simulink library "BLDC"  (Simulink 8.0)
settings: Solver=ode45  StartTime=0.0  StopTime=10.0  RelTol=1e-3
libraries: simulink x18, BLDC x1
settings Model: Creator=Juliano  LastModifiedBy=h3now

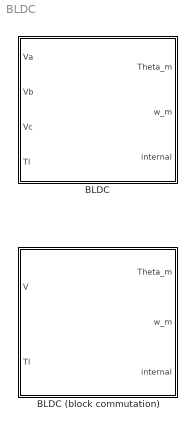
== system BLDC ==
  BLDC : Subsystem  mask(Simulador de um motor BLDC){J=1.39e-6, R=10.1/2, L=2.04/2000, P=8, Kt=15.7e-3/1.19, Ke=15.7e-3/1.19, Kd=0}
      mask prompts: J "Inércia do sistema motor+carga [Kg.m^2]"; R "Resistência por fase [Ohm]"; L "Indutância por fase [Henry]"; P "Número de pólos"; Kt "Constante de torque [Nm/A]"; Ke "Constante de força eletromotriz [V.s] (numericamente igual à constante de torque se utilizar SI)"; Kd "Constante de atrito viscoso"
      mask help:
      | Entradas
      | - Vx: tensões na fase 'x' [V]
      | - Tl: torque da carga [N.m]
      |
      | Saídas
      | - Theta_m: ângulo do rotor [rad]
      | - w_m: velocidade ângular do rotor [rad/s]
      | - internal: vetor de variáveis internas do simulador:
      |     - FCEM em cada fase [V] (3x1)
      |     - Corrente em cada fase [A] (3x1)
      |     - Torque produzido por cada fase [N.m] (3x1)
      |     - Torque total [N.m] (1x1)
  BLDC (block commutation) : Subsystem  mask(Simulador BLDC (block commutation)){J=1.39e-6, R=10.1/2, L=2.04/2000, P=8, Kt=15.7e-3/1.19, Ke=15.7e-3/1.19, Kd=0}
      mask prompts: J "Inércia do motor [Kg.m^2]"; R "Resistência por fase [Ohm]"; L "Indutância por fase [Henry]"; P "Número de pólos"; Kt "Constante de torque [Nm/A]"; Ke "Constante de força eletromotriz [V.s] (numericamente igual à constante de torque se SI)"; Kd "Constante de atrito viscoso"
      mask help:
      | Entradas
      | - Vx: tensões na fase 'x' [V]
      | - Tl: torque da carga [N.m]
      |
      | Saídas
      | - Theta_m: ângulo do rotor [rad]
      | - w_m: velocidade ângular do rotor [rad/s]
      | - internal: vetor de variáveis internas do simulador:
      |     - FCEM em cada fase [V] (3x1)
      |     - Corrente em cada fase [A] (3x1)
      |     - Torque produzido por cada fase [N.m] (3x1)
      |     - Torque total [N.m] (1x1)
      mask TypeOptions J: BLDC/J
      mask TypeOptions R: BLDC/R
      mask TypeOptions L: BLDC/L
      mask TypeOptions P: BLDC/P
      mask TypeOptions Kt: BLDC/Kt
      mask TypeOptions Ke: BLDC/Ke
      mask TypeOptions Kd: BLDC/Kd

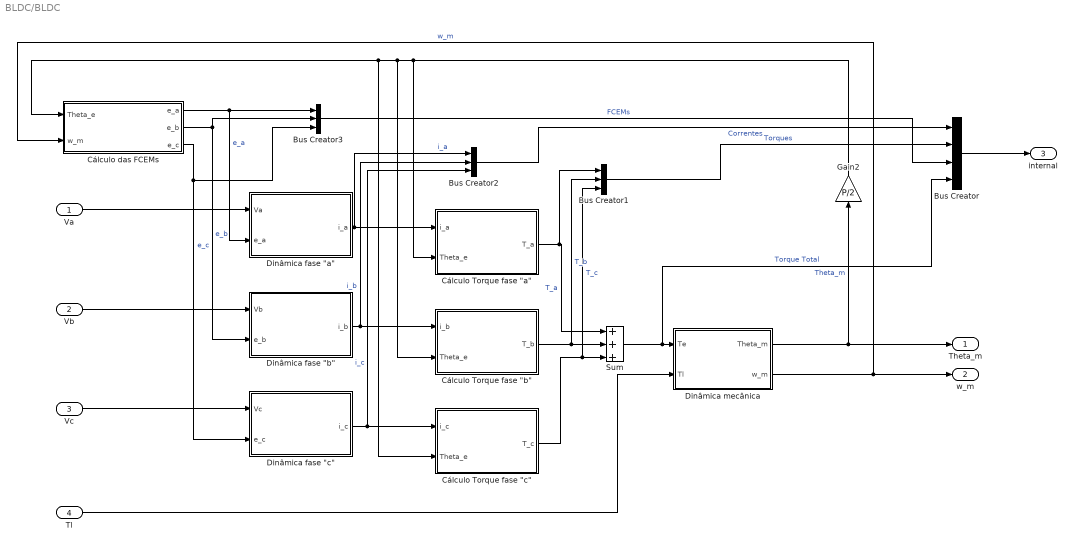
== system BLDC/BLDC ==
  Va : Inport
  Vb : Inport  Port=2
  Vc : Inport  Port=3
  Tl : Inport  Port=4
  Bus Creator : BusCreator
  Bus Creator1 : BusCreator  Inputs=3
  Bus Creator2 : BusCreator  Inputs=3
  Bus Creator3 : BusCreator  Inputs=3
  "Cálculo Torque fase \"a\"" : Subsystem
  "Cálculo Torque fase \"b\"" : Subsystem
  "Cálculo Torque fase \"c\"" : Subsystem
  Cálculo das FCEMs : Subsystem
  "Dinâmica fase \"a\"" : Subsystem
  "Dinâmica fase \"b\"" : Subsystem
  "Dinâmica fase \"c\"" : Subsystem
  "Dinâmica mecânica " : Subsystem
  Gain2 : Gain  Gain=P/2
  Sum : Sum  Inputs=+++
  Theta_m : Outport
  w_m : Outport  Port=2
  internal : Outport  Port=3
  wires:
  Gain2/1 -> "Cálculo Torque fase \"b\""/2(Theta_e), Cálculo das FCEMs/1(Theta_e), "Cálculo Torque fase \"c\""/2(Theta_e), "Cálculo Torque fase \"a\""/2(Theta_e)
  Tl/1 -> "Dinâmica mecânica "/2(Tl)
  "Dinâmica mecânica "/2(w_m) -> w_m/1, Cálculo das FCEMs/2(w_m)  "w_m"
  "Dinâmica mecânica "/1(Theta_m) -> Gain2/1, Theta_m/1  "Theta_m"
  Sum/1 -> Bus Creator/4, "Dinâmica mecânica "/1(Te)  "Torque Total"
  "Cálculo Torque fase \"c\""/1(T_c) -> Bus Creator1/3, Sum/3  "T_c"
  "Cálculo Torque fase \"b\""/1(T_b) -> Bus Creator1/2, Sum/2  "T_b"
  "Cálculo Torque fase \"a\""/1(T_a) -> Bus Creator1/1, Sum/1  "T_a"
  "Dinâmica fase \"c\""/1(i_c) -> Bus Creator2/3, "Cálculo Torque fase \"c\""/1(i_c)  "i_c"
  "Dinâmica fase \"b\""/1(i_b) -> Bus Creator2/2, "Cálculo Torque fase \"b\""/1(i_b)  "i_b"
  "Dinâmica fase \"a\""/1(i_a) -> Bus Creator2/1, "Cálculo Torque fase \"a\""/1(i_a)  "i_a"
  Vc/1 -> "Dinâmica fase \"c\""/1(Vc)
  Vb/1 -> "Dinâmica fase \"b\""/1(Vb)
  Va/1 -> "Dinâmica fase \"a\""/1(Va)
  Cálculo das FCEMs/3(e_c) -> Bus Creator3/3, "Dinâmica fase \"c\""/2(e_c)  "e_c"
  Cálculo das FCEMs/2(e_b) -> Bus Creator3/2, "Dinâmica fase \"b\""/2(e_b)  "e_b"
  Cálculo das FCEMs/1(e_a) -> Bus Creator3/1, "Dinâmica fase \"a\""/2(e_a)  "e_a"
  Bus Creator/1 -> internal/1
  Bus Creator3/1 -> Bus Creator/3  "FCEMs"
  Bus Creator2/1 -> Bus Creator/1  "Correntes"
  Bus Creator1/1 -> Bus Creator/2  "Torques"

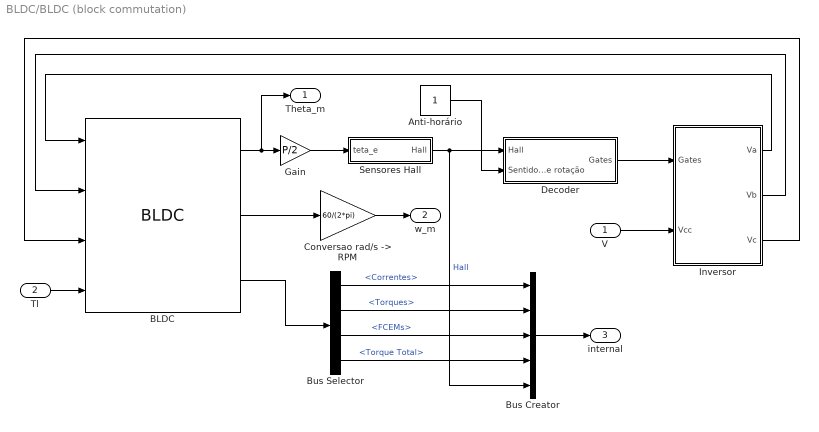
== system BLDC/BLDC (block commutation) ==
  V : Inport
  Tl : Inport  Port=2
  Anti-horário : Constant
  BLDC : BLDC/BLDC  J=J  R=R  L=L  P=P  Kt=Kt  Ke=Ke  Kd=Kd
  Bus Creator : BusCreator  Inputs=5
  Bus Selector : BusSelector  OutputSignals=Correntes,Torques,FCEMs,Torque Total
  "Conversao rad/s -> RPM" : Gain  Gain=60/(2*pi)
  Decoder : Subsystem
  Gain : Gain  Gain=P/2
  Inversor : Subsystem
  Sensores Hall : Subsystem  AncestorBlock=spsPMSynchronousMachineModel/Discrete Trapezoidal/Hall effect sensor
  Theta_m : Outport
  w_m : Outport  Port=2
  internal : Outport  Port=3
  wires:
  BLDC/1 -> Theta_m/1, Gain/1
  Gain/1 -> Sensores Hall/1(teta_e)
  Decoder/1(Gates) -> Inversor/1(Gates)
  Anti-horário/1 -> Decoder/2(Sentido de rotação)
  Tl/1 -> BLDC/4
  Inversor/1(Va) -> BLDC/1
  Inversor/2(Vb) -> BLDC/2
  Inversor/3(Vc) -> BLDC/3
  BLDC/2 -> "Conversao rad/s -> RPM"/1
  "Conversao rad/s -> RPM"/1 -> w_m/1
  V/1 -> Inversor/2(Vcc)
  Sensores Hall/1(Hall) -> Bus Creator/5, Decoder/1("Hall ")  "Hall"
  BLDC/3 -> Bus Selector/1
  Bus Selector/1 -> Bus Creator/1  "<Correntes>"
  Bus Selector/2 -> Bus Creator/2  "<Torques>"
  Bus Selector/3 -> Bus Creator/3  "<FCEMs>"
  Bus Selector/4 -> Bus Creator/4  "<Torque Total>"
  Bus Creator/1 -> internal/1

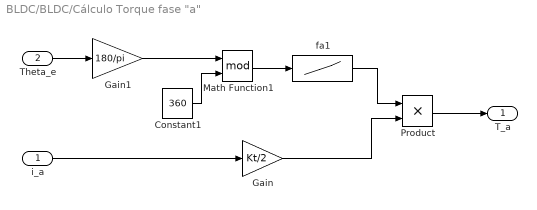
== system BLDC/BLDC/Cálculo Torque fase "a" ==
  i_a : Inport
  Theta_e : Inport  Port=2
  Constant1 : Constant  Value=360
  Gain : Gain  Gain=Kt/2
  Gain1 : Gain  Gain=180/pi
  Math Function1 : Math  Operator=mod  SaturateOnIntegerOverflow=on
  Product : Product  RndMeth=Zero
  fa1 : Lookup  InputValues=[0 30 60 90 120 150 180 210 240 270 300 330 360]  Table=[ 1 1 1 0 -1 -1 -1 -1 -1 0 1 1 1]
  T_a : Outport
  wires:
  Constant1/1 -> Math Function1/2
  Gain1/1 -> Math Function1/1
  Product/1 -> T_a/1
  fa1/1 -> Product/1
  Theta_e/1 -> Gain1/1
  Math Function1/1 -> fa1/1
  Gain/1 -> Product/2
  i_a/1 -> Gain/1

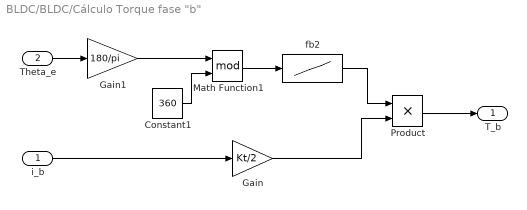
== system BLDC/BLDC/Cálculo Torque fase "b" ==
  i_b : Inport
  Theta_e : Inport  Port=2
  Constant1 : Constant  Value=360
  Gain : Gain  Gain=Kt/2
  Gain1 : Gain  Gain=180/pi
  Math Function1 : Math  Operator=mod  SaturateOnIntegerOverflow=on
  Product : Product  RndMeth=Zero
  fb2 : Lookup  InputValues=[0 30 60 90 120 150 180 210 240 270 300 330 360]  Table=[-1 0 1 1 1 1 1 0 -1 -1 -1 -1 -1]
  T_b : Outport
  wires:
  Constant1/1 -> Math Function1/2
  Gain1/1 -> Math Function1/1
  i_b/1 -> Gain/1
  Gain/1 -> Product/2
  Math Function1/1 -> fb2/1
  Theta_e/1 -> Gain1/1
  fb2/1 -> Product/1
  Product/1 -> T_b/1

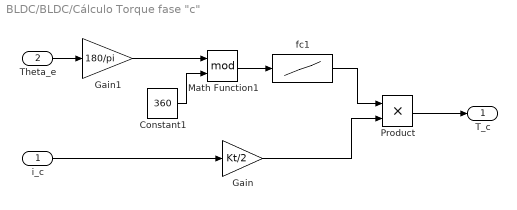
== system BLDC/BLDC/Cálculo Torque fase "c" ==
  i_c : Inport
  Theta_e : Inport  Port=2
  Constant1 : Constant  Value=360
  Gain : Gain  Gain=Kt/2
  Gain1 : Gain  Gain=180/pi
  Math Function1 : Math  Operator=mod  SaturateOnIntegerOverflow=on
  Product : Product  RndMeth=Zero
  fc1 : Lookup  InputValues=[0 30 60 90 120 150 180 210 240 270 300 330 360]  Table=[-1 -1 -1 -1 -1 0 1 1 1 1 1 0 -1]
  T_c : Outport
  wires:
  Constant1/1 -> Math Function1/2
  Gain1/1 -> Math Function1/1
  Product/1 -> T_c/1
  fc1/1 -> Product/1
  Theta_e/1 -> Gain1/1
  Math Function1/1 -> fc1/1
  Gain/1 -> Product/2
  i_c/1 -> Gain/1

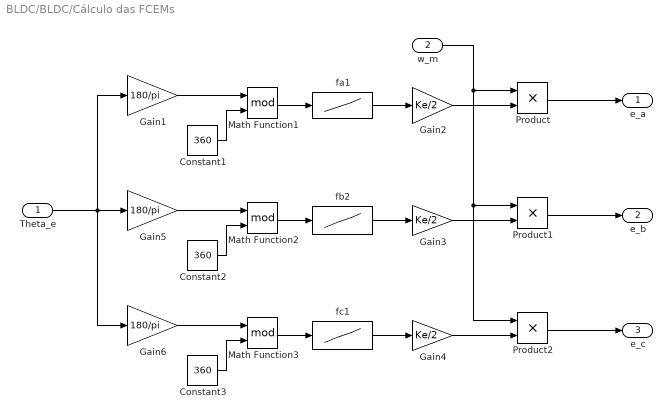
== system BLDC/BLDC/Cálculo das FCEMs ==
  Theta_e : Inport
  w_m : Inport  Port=2
  Constant1 : Constant  Value=360
  Constant2 : Constant  Value=360
  Constant3 : Constant  Value=360
  Gain1 : Gain  Gain=180/pi
  Gain2 : Gain  Gain=Ke/2
  Gain3 : Gain  Gain=Ke/2
  Gain4 : Gain  Gain=Ke/2
  Gain5 : Gain  Gain=180/pi
  Gain6 : Gain  Gain=180/pi
  Math Function1 : Math  Operator=mod  SaturateOnIntegerOverflow=on
  Math Function2 : Math  Operator=mod  SaturateOnIntegerOverflow=on
  Math Function3 : Math  Operator=mod  SaturateOnIntegerOverflow=on
  Product : Product  RndMeth=Zero
  Product1 : Product  RndMeth=Zero
  Product2 : Product  RndMeth=Zero
  fa1 : Lookup  InputValues=[0 30 60 90 120 150 180 210 240 270 300 330 360]  Table=[ 1 1 1 0 -1 -1 -1 -1 -1 0 1 1 1]
  fb2 : Lookup  InputValues=[0 30 60 90 120 150 180 210 240 270 300 330 360]  Table=[-1 0 1 1 1 1 1 0 -1 -1 -1 -1 -1]
  fc1 : Lookup  InputValues=[0 30 60 90 120 150 180 210 240 270 300 330 360]  Table=[-1 -1 -1 -1 -1 0 1 1 1 1 1 0 -1]
  e_a : Outport
  e_b : Outport  Port=2
  e_c : Outport  Port=3
  wires:
  Constant3/1 -> Math Function3/2
  Constant2/1 -> Math Function2/2
  Constant1/1 -> Math Function1/2
  Product/1 -> e_a/1
  Product1/1 -> e_b/1
  Theta_e/1 -> Gain5/1, Gain1/1, Gain6/1
  Product2/1 -> e_c/1
  Gain2/1 -> Product/2
  w_m/1 -> Product/1, Product1/1, Product2/1
  Gain3/1 -> Product1/2
  Gain4/1 -> Product2/2
  Gain1/1 -> Math Function1/1
  Gain5/1 -> Math Function2/1
  Gain6/1 -> Math Function3/1
  Math Function1/1 -> fa1/1
  fa1/1 -> Gain2/1
  Math Function2/1 -> fb2/1
  fb2/1 -> Gain3/1
  Math Function3/1 -> fc1/1
  fc1/1 -> Gain4/1

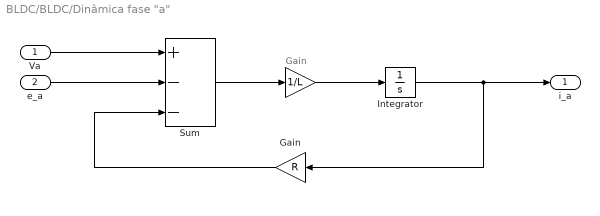
== system BLDC/BLDC/Dinâmica fase "a" ==
  note: Gain
  Va : Inport
  e_a : Inport  Port=2
  " " : Gain  Gain=1/L
  Gain : Gain  Gain=R
  Integrator : Integrator
  Sum : Sum  Inputs=+--
  i_a : Outport
  wires:
  e_a/1 -> Sum/2
  Gain/1 -> Sum/3
  " "/1 -> Integrator/1
  Sum/1 -> " "/1
  Va/1 -> Sum/1
  Integrator/1 -> Gain/1, i_a/1

== system BLDC/BLDC/Dinâmica fase "b" ==
  note: Gain
  Vb : Inport
  e_b : Inport  Port=2
  " " : Gain  Gain=1/L
  Gain : Gain  Gain=R
  Integrator : Integrator
  Sum : Sum  Inputs=+--
  i_b : Outport
  wires:
  Integrator/1 -> i_b/1, Gain/1
  Vb/1 -> Sum/1
  Sum/1 -> " "/1
  " "/1 -> Integrator/1
  Gain/1 -> Sum/3
  e_b/1 -> Sum/2

== system BLDC/BLDC/Dinâmica fase "c" ==
  note: Gain
  Vc : Inport
  e_c : Inport  Port=2
  " " : Gain  Gain=1/L
  Gain : Gain  Gain=R
  Integrator : Integrator
  Sum : Sum  Inputs=+--
  i_c : Outport
  wires:
  e_c/1 -> Sum/2
  Gain/1 -> Sum/3
  " "/1 -> Integrator/1
  Sum/1 -> " "/1
  Vc/1 -> Sum/1
  Integrator/1 -> Gain/1, i_c/1

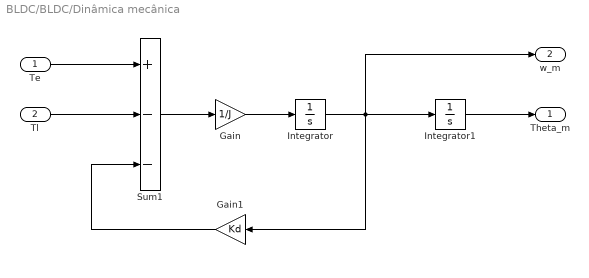
== system BLDC/BLDC/Dinâmica mecânica  ==
  Te : Inport
  Tl : Inport  Port=2
  Gain : Gain  Gain=1/J
  Gain1 : Gain  Gain=Kd
  Integrator : Integrator
  Integrator1 : Integrator
  Sum1 : Sum  Inputs=+--
  Theta_m : Outport
  w_m : Outport  Port=2
  wires:
  Integrator1/1 -> Theta_m/1
  Tl/1 -> Sum1/2
  Gain1/1 -> Sum1/3
  Te/1 -> Sum1/1
  Integrator/1 -> Gain1/1, Integrator1/1, w_m/1
  Gain/1 -> Integrator/1
  Sum1/1 -> Gain/1

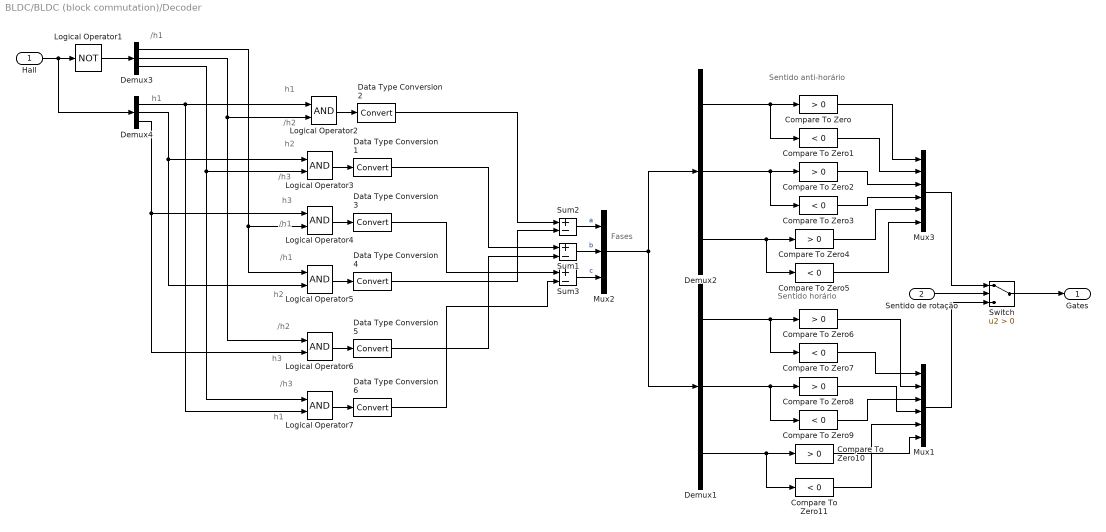
== system BLDC/BLDC (block commutation)/Decoder ==
  note: Fases
  note: Sentido horário
  note: Sentido anti-horário
  note: h1
  note: /h3
  note: h3
  note: /h2
  note: h2
  note: /h1
  note: /h1
  note: h3
  note: /h3
  note: h2
  note: /h2
  note: h1
  note: h1
  note: /h1
  "Hall " : Inport
  Sentido de rotação : Inport  Port=2
  Compare To Zero{,2,4,6,8,10} (6 alike) : simulink/Logic and Bit Operations/Compare To Zero  relop=>  OutDataTypeStr=boolean  ZeroCross=off
  Compare To Zero{1,3,5,7,9,11} (6 alike) : simulink/Logic and Bit Operations/Compare To Zero  relop=<  OutDataTypeStr=boolean  ZeroCross=off
  Data Type Conversion{1..6} (6 alike) : DataTypeConversion
  Demux{1..4} (4 alike) : Demux  Outputs=3
  Logical Operator1 : Logic  Operator=NOT  AllPortsSameDT=off  OutDataTypeStr=boolean
  Logical Operator{2..7} (6 alike) : Logic  AllPortsSameDT=off  OutDataTypeStr=boolean
  Mux1 : Mux  Inputs=6
  Mux2 : Mux  Inputs=3
  Mux3 : Mux  Inputs=6
  Sum1 : Sum  Inputs=+-  OutDataTypeStr=double
  Sum2 : Sum  Inputs=+-  OutDataTypeStr=double
  Sum3 : Sum  Inputs=+-  OutDataTypeStr=double
  Switch : Switch  Criteria=u2 > Threshold
  Gates : Outport
  wires:
  Mux2/1 -> Demux1/1, Demux2/1
  Data Type Conversion6/1 -> Sum3/2
  Data Type Conversion3/1 -> Sum3/1
  Data Type Conversion5/1 -> Sum1/2
  Data Type Conversion1/1 -> Sum1/1
  Data Type Conversion4/1 -> Sum2/2
  Data Type Conversion2/1 -> Sum2/1
  Logical Operator7/1 -> Data Type Conversion6/1
  Logical Operator6/1 -> Data Type Conversion5/1
  Logical Operator5/1 -> Data Type Conversion4/1
  Logical Operator4/1 -> Data Type Conversion3/1
  Logical Operator3/1 -> Data Type Conversion1/1
  Sum3/1 -> Mux2/3  "c"
  Sum1/1 -> Mux2/2  "b"
  Sum2/1 -> Mux2/1  "a"
  Logical Operator2/1 -> Data Type Conversion2/1
  Demux3/1 -> Logical Operator5/1, Logical Operator4/2
  Demux3/2 -> Logical Operator6/1, Logical Operator2/2
  Demux3/3 -> Logical Operator7/1, Logical Operator3/2
  Demux4/1 -> Logical Operator7/2, Logical Operator2/1
  Demux4/2 -> Logical Operator5/2, Logical Operator3/1
  Demux4/3 -> Logical Operator6/2, Logical Operator4/1
  Logical Operator1/1 -> Demux3/1
  "Hall "/1 -> Demux4/1, Logical Operator1/1
  Compare To Zero10/1 -> Mux1/6
  Compare To Zero11/1 -> Mux1/5
  Compare To Zero8/1 -> Mux1/4
  Compare To Zero9/1 -> Mux1/3
  Compare To Zero6/1 -> Mux1/2
  Compare To Zero7/1 -> Mux1/1
  Switch/1 -> Gates/1
  Mux1/1 -> Switch/3
  Sentido de rotação/1 -> Switch/2
  Mux3/1 -> Switch/1
  Demux1/3 -> Compare To Zero11/1, Compare To Zero10/1
  Demux1/2 -> Compare To Zero9/1, Compare To Zero8/1
  Demux1/1 -> Compare To Zero7/1, Compare To Zero6/1
  Compare To Zero5/1 -> Mux3/6
  Compare To Zero4/1 -> Mux3/5
  Compare To Zero3/1 -> Mux3/4
  Compare To Zero2/1 -> Mux3/3
  Compare To Zero1/1 -> Mux3/2
  Compare To Zero/1 -> Mux3/1
  Demux2/3 -> Compare To Zero5/1, Compare To Zero4/1
  Demux2/2 -> Compare To Zero3/1, Compare To Zero2/1
  Demux2/1 -> Compare To Zero1/1, Compare To Zero/1

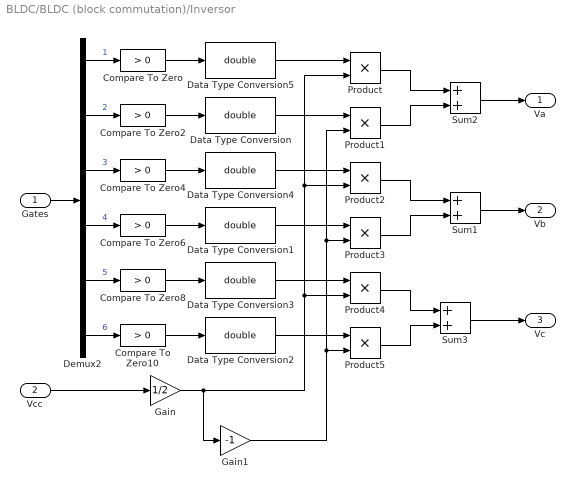
== system BLDC/BLDC (block commutation)/Inversor ==
  Gates : Inport
  Vcc : Inport  Port=2
  Compare To Zero : simulink/Logic and Bit Operations/Compare To Zero  relop=>  OutDataTypeStr=uint8  ZeroCross=off
  Compare To Zero{2,6,8,10} (4 alike) : simulink/Logic and Bit Operations/Compare To Zero  relop=>  OutDataTypeStr=boolean  ZeroCross=off
  Compare To Zero4 : simulink/Logic and Bit Operations/Compare To Zero  relop=>  OutDataTypeStr=uint8  ZeroCross=off
  Data Type Conversion{,1..5} (6 alike) : DataTypeConversion  OutDataTypeStr=double
  Demux2 : Demux  Outputs=6
  Gain : Gain  Gain=1/2
  Gain1 : Gain  Gain=-1
  Product{,1..5} (6 alike) : Product  RndMeth=Zero
  Sum1 : Sum  SaturateOnIntegerOverflow=on
  Sum2 : Sum  SaturateOnIntegerOverflow=on
  Sum3 : Sum  SaturateOnIntegerOverflow=on
  Va : Outport
  Vb : Outport  Port=2
  Vc : Outport  Port=3
  wires:
  Vcc/1 -> Gain/1
  Sum1/1 -> Vb/1
  Sum3/1 -> Vc/1
  Sum2/1 -> Va/1
  Gates/1 -> Demux2/1
  Demux2/1 -> Compare To Zero/1  "1"
  Demux2/2 -> Compare To Zero2/1  "2"
  Demux2/3 -> Compare To Zero4/1  "3"
  Demux2/4 -> Compare To Zero6/1  "4"
  Demux2/5 -> Compare To Zero8/1  "5"
  Demux2/6 -> Compare To Zero10/1  "6"
  Compare To Zero/1 -> Data Type Conversion5/1
  Compare To Zero2/1 -> Data Type Conversion/1
  Compare To Zero4/1 -> Data Type Conversion4/1
  Compare To Zero6/1 -> Data Type Conversion1/1
  Compare To Zero8/1 -> Data Type Conversion3/1
  Compare To Zero10/1 -> Data Type Conversion2/1
  Product/1 -> Sum2/1
  Product1/1 -> Sum2/2
  Product2/1 -> Sum1/1
  Product3/1 -> Sum1/2
  Product4/1 -> Sum3/1
  Product5/1 -> Sum3/2
  Data Type Conversion2/1 -> Product5/1
  Data Type Conversion3/1 -> Product4/1
  Data Type Conversion1/1 -> Product3/1
  Data Type Conversion4/1 -> Product2/1
  Data Type Conversion/1 -> Product1/1
  Data Type Conversion5/1 -> Product/1
  Gain1/1 -> Product5/2, Product3/2, Product1/2
  Gain/1 -> Gain1/1, Product4/2, Product2/2, Product/2

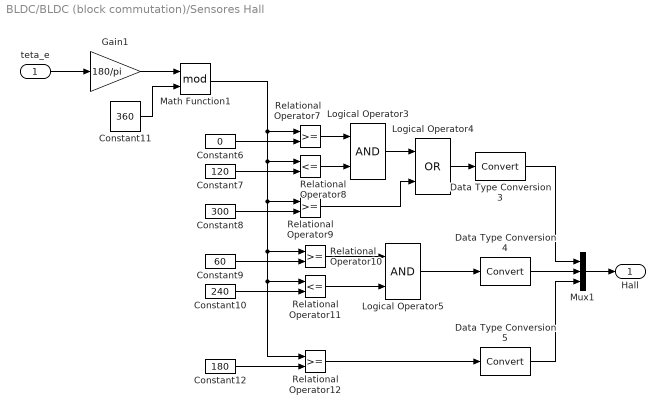
== system BLDC/BLDC (block commutation)/Sensores Hall ==
  teta_e : Inport
  Constant10 : Constant  Value=240
  Constant11 : Constant  Value=360
  Constant12 : Constant  Value=180
  Constant6 : Constant  Value=0
  Constant7 : Constant  Value=120
  Constant8 : Constant  Value=300
  Constant9 : Constant  Value=60
  Data Type Conversion3 : DataTypeConversion  SaturateOnIntegerOverflow=on  RndMeth=Zero
  Data Type Conversion4 : DataTypeConversion  SaturateOnIntegerOverflow=on  RndMeth=Zero
  Data Type Conversion5 : DataTypeConversion  SaturateOnIntegerOverflow=on  RndMeth=Zero
  Gain1 : Gain  Gain=180/pi
  Logical Operator3 : Logic  AllPortsSameDT=off  OutDataTypeStr=boolean
  Logical Operator4 : Logic  Operator=OR  AllPortsSameDT=off  OutDataTypeStr=boolean
  Logical Operator5 : Logic  AllPortsSameDT=off  OutDataTypeStr=boolean
  Math Function1 : Math  Operator=mod  SaturateOnIntegerOverflow=on
  Mux1 : Mux  Inputs=3
  Relational Operator{7,9..10,12} (4 alike) : RelationalOperator  InputSameDT=on
  Relational Operator11 : RelationalOperator  Operator=<=  InputSameDT=on
  Relational Operator8 : RelationalOperator  Operator=<=  InputSameDT=on
  Hall : Outport
  wires:
  teta_e/1 -> Gain1/1
  Constant6/1 -> Relational Operator7/2
  Constant7/1 -> Relational Operator8/2
  Constant8/1 -> Relational Operator9/2
  Relational Operator9/1 -> Logical Operator4/2
  Logical Operator3/1 -> Logical Operator4/1
  Relational Operator7/1 -> Logical Operator3/1
  Relational Operator8/1 -> Logical Operator3/2
  Relational Operator10/1 -> Logical Operator5/1
  Relational Operator11/1 -> Logical Operator5/2
  Constant9/1 -> Relational Operator10/2
  Constant10/1 -> Relational Operator11/2
  Constant12/1 -> Relational Operator12/2
  Mux1/1 -> Hall/1
  Data Type Conversion3/1 -> Mux1/1
  Data Type Conversion4/1 -> Mux1/2
  Data Type Conversion5/1 -> Mux1/3
  Logical Operator4/1 -> Data Type Conversion3/1
  Logical Operator5/1 -> Data Type Conversion4/1
  Relational Operator12/1 -> Data Type Conversion5/1
  Gain1/1 -> Math Function1/1
  Constant11/1 -> Math Function1/2
  Math Function1/1 -> Relational Operator8/1, Relational Operator9/1, Relational Operator10/1, Relational Operator11/1, Relational Operator12/1, Relational Operator7/1
